simulink model "VectorControl003"  (R2019b)
settings: Solver=ode15s  StartTime=0  StopTime=1  FixedStep=0.001  MaxStep=1e-4  RelTol=1e-6  AbsTol=1e-6  EnableMultiTasking=on
StopFcn:
  | % TNAnalyzexxxPlot
values from neighbouring files (symbols this model uses):
  CurGainError_U = 1 + 0.2*(rand() - 0.5)    [Param000.m]    (also in StartSim.m)
  CurGainError_V = 1 + 0.2*(rand() - 0.5)    [Param000.m]    (also in StartSim.m)
  CurGainError_W = 1 + 0.2*(rand() - 0.5)    [Param000.m]    (also in StartSim.m)
  CurOfsError_U = 0.5 * rand()    [Param000.m]    (also in StartSim.m = AmpNoise * rand())
  CurOfsError_V = 0.5 * rand()    [Param000.m]    (also in StartSim.m = AmpNoise * rand())
  CurOfsError_W = 0.5 * rand()    [Param000.m]    (also in StartSim.m = AmpNoise * rand())
  DCVoltage = 100    [Param000.m]    (also in StartSim.m; StartSim_NoNoise.m)
  ElecAngOfsError = pi*2.0*(rand() - 0.5)    [Param000.m]    (also in StartSim.m = pi * 2.0 * (rand() - 0.5); StartSim_NoNoise.m = pi * 2.0 * (rand() - 0.5))
  MotInertia = 10*rand()*1e-3    [Param000.m]    (also in StartSim.m = 0.1*rand()*1e-3; StartSim_NoNoise.m = 0.1*rand()*1e-3)
  MotPhaseL = 38.7e-6    (= 3.87e-05)    [Param000.m]    (also in StartSim.m = (0.001 + 10 * rand())*1e-3; StartSim_NoNoise.m = (0.001 + 10 * rand())*1e-3)
  MotPhaseR = 25e-3    (= 0.025)    [Param000.m]    (also in StartSim.m = 0.001 + 10 * rand(); StartSim_NoNoise.m = 0.001 + 10 * rand())
  MotPole = 20    [Param000.m]    (also in StartSim.m = 1; StartSim_NoNoise.m = 1)
  MotVisco = rand()*1e-6    [Param000.m]    (also in StartSim.m = 0.01*rand()*1e-6; StartSim_NoNoise.m = 0.01*rand()*1e-6)
  Ts = 1e-6    (= 1e-06)    [StartSim.m]    (also in StartSim_NoNoise.m)
libraries: powerlib x16, simulink x4, powerlib_meascontrol x2, eePwmGeneratorTwoLevel x1
Description:
  | This example illustrates use of the BLDC in a closed-loop
  | speed and voltage control on a 1 kW, 3000 rpm industrial motor
  | 
  | 
  | Copyright 2008-2017 The MathWorks, Inc.
settings Model: ExtModeAutoUpdateStatusClock=off  Creator=MathWorks  LastModifiedBy=nb1e4
settings SolverCC: AutoScaleAbsTol=off  MaxConsecutiveZCs=10000  ZeroCrossAlgorithm=Adaptive  DecoupledContinuousIntegration=on
settings DataIOCC: Decimation=100  SaveFormat=Array  SignalLoggingName=sigsOut
settings OptimizationCC: DefaultParameterBehavior=Inlined  UseDivisionForNetSlopeComputation=on  UseFloatMulNetSlope=on  InlineInvariantSignals=on  PassReuseOutputArgsAs=Individual arguments  ExpressionDepthLimit=2147483647  ZeroExternalMemoryAtStartup=off  ZeroInternalMemoryAtStartup=off  NoFixptDivByZeroProtection=on  EfficientFloat2IntCast=on  LifeSpan=1  OptimizeDataStoreBuffers=off  BusAssignmentInplaceUpdate=off  OptimizationLevel=level0  EfficientTunableParamExpr=on
settings DebuggingCC: AlgebraicLoopMsg=none  UnderspecifiedInitializationDetection=Classic  MergeDetectMultiDrivingBlocksExec=none  SignalResolutionControl=TryResolveAllWithWarning  MultiTaskDSMMsg=warning  MultiTaskCondExecSysMsg=none  ParameterTunabilityLossMsg=error  FcnCallInpInsideContextMsg=warning  StateNameClashWarn=warning  SFUnexpectedBacktrackingDiag=warning  SFNoUnconditionalDefaultTransitionDiag=warning  SFExecutionAtInitializationDiag=none  ArithmeticOperatorsInVariantConditions=warning
settings HardwareCC: ProdBitPerPointer=32  ProdBitPerSizeT=32  ProdBitPerPtrDiffT=32  ProdLargestAtomicInteger=Long  ProdWordSize=32  ProdLongLongMode=on  ProdHWDeviceType=ARM Compatible->ARM 10  TargetUnknown=on
settings ModelReferenceCC: PropagateSignalLabelsOutOfModel=off
settings SFSimCC: SimUseLocalCustomCode=off  MATLABDynamicMemAlloc=off  CustomCodeUndefinedFunction=UseInterfaceOnly
settings RTWCC: SystemTargetFile=ert.tlc  TemplateMakefile=ert_default_tmf  GenerateReport=on  RTWUseLocalCustomCode=off  IncludeHyperlinkInReport=on  LaunchReport=on  GenerateTraceInfo=on  GenerateTraceReport=on  GenerateTraceReportSl=on  GenerateTraceReportSf=on  GenerateTraceReportEml=on  GenerateCodeMetricsReport=on
settings CodeAppCC: ForceParamTrailComments=on  IgnoreCustomStorageClasses=off  OperatorAnnotations=on  SimulinkDataObjDesc=on  SFDataObjDesc=on  CustomSymbolStrGlobalVar=rt$N$M  CustomSymbolStrType=$N$M  CustomSymbolStrFcn=$N$M$F  CustomSymbolStrMacro=$N$M  InsertBlockDesc=on
settings ERTTargetCC: GenerateSampleERTMain=on  IncludeMdlTerminateFcn=off  CombineSignalStateStructs=on  SupportComplex=off  SupportContinuousTime=on  SupportNonInlinedSFcns=on  InlinedParameterPlacement=NonHierarchical  ERTCustomFileTemplate=example_file_process.tlc  ERTFilePackagingFormat=CompactWithDataFile
settings ConfigComp: CovMetricSettings=dw  CovHtmlReporting=on  CovSaveCumulativeToWorkspaceVar=on  CovSaveSingleToWorkspaceVar=on  CovExternalEMLEnable=off  CovSFcnEnable=off
settings SimscapeCC: SimscapeNormalizeSystem=off

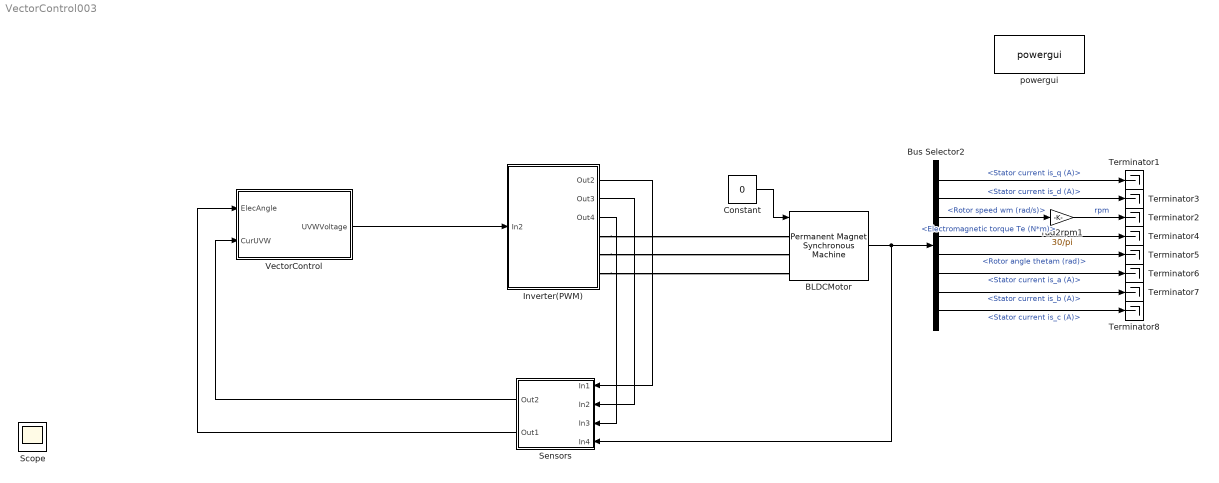
== system VectorControl003 ==
  BLDCMotor : powerlib/Machines/Permanent Magnet Synchronous Machine  NbPhases=3  FluxDistribution=Sinusoidal  RotorType=Round  MechanicalLoad=Torque Tm  PresetModel=No  ShowDetailedParameters=on  MeasurementBus=off  Resistance=MotPhaseR  Inductance=MotPhaseL  dqInductances=[8.5e-3, 8.5e-3]  La=MotPhaseL  MachineConstant=Voltage Constant (V_peak L-L / krpm)  Flux=0.01021  VoltageCst=MotVoltageConst  TorqueCst=0.30629  Flat=120  Mechanical=[MotInertia MotVisco MotPole 0]  PolePairs=20  InitialConditions=[0,0, 0,0]  InitialConditions5ph=[0 0 0 0 0 0]  RefAngle=90 degrees behind phase A axis (modified Park)  IterativeDiscreteModel=Trapezoidal non iterative  TsBlock=-1  TsPowergui=0
  Bus Selector2 : BusSelector  OutputSignals=Stator current is_q (A),Stator current is_d (A),Rotor speed wm (rad/s),Electromagnetic torque Te (N*m),Rotor angle thetam (rad),Stator current is_a (A),Stator current is_b (A),Stator current is_c (A)
  Constant : Constant  Value=0
  Inverter(PWM) : Subsystem
  Sensors : Subsystem
  Terminator{1..8} (8 alike) : Terminator
  VectorControl : Subsystem
  powergui : powerlib/powergui  Priority=2  SimulationMode=Continuous  SampleTime=Ts  frequency=60  Iterations=50  frequencyindice=0  Pbase=100e6  ErrMax=1e-4  UnitsV=kV  UnitsW=MW  buscounter=0  FunctionMessages=off  echomessages=off  EnableUseOfTLC=off  CurrentSourceSwitches=off  DisableSnubberDevices=off  DisableRonSwitches=off  DisableVfSwitches=off  DisplayEquations=off  AutomaticDiscreteSolvers=off  SolverType=Tustin/Backward Euler (TBE)  Interpol=off  ExternalGateDelay=off  methode=off  Ts=100  x0status=blocks  SPID=off  SwTol=0  HookPort=off  NonlinearTolerance=1e-4  nMaxIteration=100  ContinueOnMaxIteration=off  RestoreLinks=warning  ResistiveCurrentMeasurement=off  Frange=[0:2:500]  Ylog=off  Xlog=on  ShowGrid=off  save=off  variable=ZData  structure=0  ZoomFFT=on  StartTime=0.0  cycles=1  DisplayStyle=1  fundamental=60  FreqAxis=off  MaxFrequency=1000  frequencyindicesteady=1  RmsSteady=1  display=off
      settings: SourceProductName=Simscape Electrical
  rad2rpm1 : Gain  Gain=30/pi
  Scope : Scope
  wires:
  Bus Selector2/3 -> rad2rpm1/1  "<Rotor speed wm (rad/s)>"
  BLDCMotor/1 -> Sensors/4(In4), Bus Selector2/1
  rad2rpm1/1 -> Terminator2/1  "rpm"
  Bus Selector2/1 -> Terminator1/1  "<Stator current is_q (A)>"
  Bus Selector2/2 -> Terminator3/1  "<Stator current is_d (A)>"
  Bus Selector2/4 -> Terminator4/1  "<Electromagnetic torque Te (N*m)>"
  Bus Selector2/5 -> Terminator5/1  "<Rotor angle thetam (rad)>"
  Bus Selector2/6 -> Terminator6/1  "<Stator current is_a (A)>"
  Bus Selector2/7 -> Terminator7/1  "<Stator current is_b (A)>"
  Bus Selector2/8 -> Terminator8/1  "<Stator current is_c (A)>"
  Inverter(PWM)/1(Out2) -> Sensors/1(In1)
  Inverter(PWM)/2(Out3) -> Sensors/2(In2)
  Inverter(PWM)/3(Out4) -> Sensors/3(In3)
  VectorControl/1(UVWVoltage) -> Inverter(PWM)/1(In2)
  Sensors/1(Out2) -> VectorControl/2(CurUVW)
  Sensors/2(Out1) -> VectorControl/1(ElecAngle)
  Constant/1 -> BLDCMotor/1
  connections:
  Inverter(PWM)/RConn2 -- BLDCMotor/LConn2
  Inverter(PWM)/RConn3 -- BLDCMotor/LConn3
  Inverter(PWM)/RConn1 -- BLDCMotor/LConn1

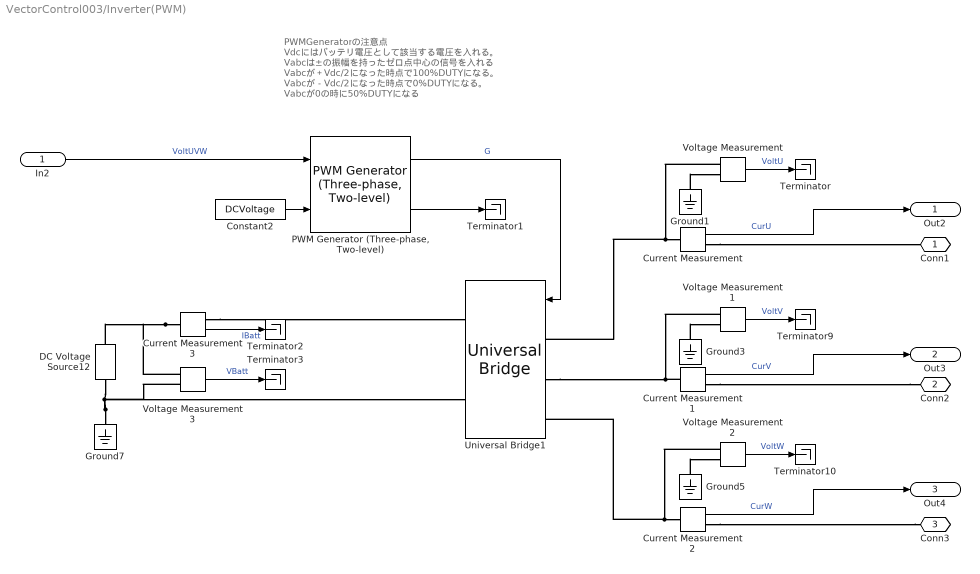
== system VectorControl003/Inverter(PWM) ==
  note: PWMGeneratorの注意点
      | Vdcにはバッテリ電圧として該当する電圧を入れる。
      | Vabcは±の振幅を持ったゼロ点中心の信号を入れる
      | Vabcが＋Vdc/2になった時点で100%DUTYになる。
      | Vabcが－Vdc/2になった時点で0%DUTYになる。
      | Vabcが0の時に50%DUTYになる
  In2 : Inport
  Constant2 : Constant  Value=DCVoltage
  Current Measurement{,1..3} (4 alike) : powerlib/Measurements/Current Measurement  PhasorSimulation=off  OutputType=Complex  PSBequivalent=0
      settings: SourceProductName=Simscape Electrical
  DC Voltage Source12 : powerlib/Electrical Sources/DC Voltage Source  Amplitude=DCVoltage  Measurements=None
      settings: SourceProductName=Simscape Electrical
  Ground{1,3,5,7} (4 alike) : powerlib/Elements/Ground  LConnTagsString=a
      settings: SourceProductName=Simscape Electrical
  "PWM Generator (Three-phase, Two-level)" : eePwmGeneratorTwoLevel/PWM Generator (Three-phase, Two-level)  PWMMode=Continuous PWM (CPWM)  CPWMMode=SPWM: sinusoidal PWM  DPWMMode=60 DPWM: 60 degree discontinuous PWM  fsw=AmpCarryFreq  Ts=1e-6
      settings: SourceProductName=Simscape Electrical  SourceProductBaseCode=PS
  Terminator{,1..3,9..10} (6 alike) : Terminator
  Universal Bridge1 : powerlib/Power Electronics/Universal Bridge  Arms=3  SnubberResistance=1e5  SnubberCapacitance=inf  Device=MOSFET / Diodes  Ron=1e-6  Lon=0  ForwardVoltages="[  0  0  ]"  ForwardVoltage=0  GTOparameters=[ 10e-6 , 20e-6 ]  IGBTparameters=[ 1e-6 , 2e-6 ]  Measurements=None  Measurements_2=None  converterType=Rectifier
      settings: SourceProductName=Simscape Electrical
  Voltage Measurement{,1..3} (4 alike) : powerlib/Measurements/Voltage Measurement  PhasorSimulation=off  OutputType=Complex  PSBequivalent=0
      settings: SourceProductName=Simscape Electrical
  Conn1 : PMIOPort  Side=Right
  Conn2 : PMIOPort  Port=2  Side=Right
  Conn3 : PMIOPort  Port=3  Side=Right
  Out2 : Outport  VectorParamsAs1DForOutWhenUnconnected=off
  Out3 : Outport  Port=2  VectorParamsAs1DForOutWhenUnconnected=off
  Out4 : Outport  Port=3  VectorParamsAs1DForOutWhenUnconnected=off
  wires:
  Voltage Measurement1/1 -> Terminator9/1  "VoltV"
  Voltage Measurement2/1 -> Terminator10/1  "VoltW"
  Voltage Measurement/1 -> Terminator/1  "VoltU"
  Current Measurement1/1 -> Out3/1  "CurV"
  Current Measurement2/1 -> Out4/1  "CurW"
  Current Measurement/1 -> Out2/1  "CurU"
  Current Measurement3/1 -> Terminator2/1  "IBatt"
  Voltage Measurement3/1 -> Terminator3/1  "VBatt"
  Constant2/1 -> "PWM Generator (Three-phase, Two-level)"/2
  "PWM Generator (Three-phase, Two-level)"/1 -> Universal Bridge1/1  "G"
  "PWM Generator (Three-phase, Two-level)"/2 -> Terminator1/1
  In2/1 -> "PWM Generator (Three-phase, Two-level)"/1  "VoltUVW"
  connections:
  Voltage Measurement/LConn1 -- Current Measurement/LConn1 -- Universal Bridge1/LConn1
  Voltage Measurement2/LConn1 -- Current Measurement2/LConn1 -- Universal Bridge1/LConn3
  Current Measurement1/LConn1 -- Voltage Measurement1/LConn1 -- Universal Bridge1/LConn2
  Ground1/LConn1 -- Voltage Measurement/LConn2
  Ground3/LConn1 -- Voltage Measurement1/LConn2
  Ground5/LConn1 -- Voltage Measurement2/LConn2
  Current Measurement3/LConn1 -- Voltage Measurement3/LConn1 -- DC Voltage Source12/RConn1
  Ground7/LConn1 -- Universal Bridge1/RConn2 -- Voltage Measurement3/LConn2 -- DC Voltage Source12/LConn1
  Current Measurement/RConn1 -- Conn1/RConn1
  Current Measurement1/RConn1 -- Conn2/RConn1
  Current Measurement2/RConn1 -- Conn3/RConn1
  Current Measurement3/RConn1 -- Universal Bridge1/RConn1

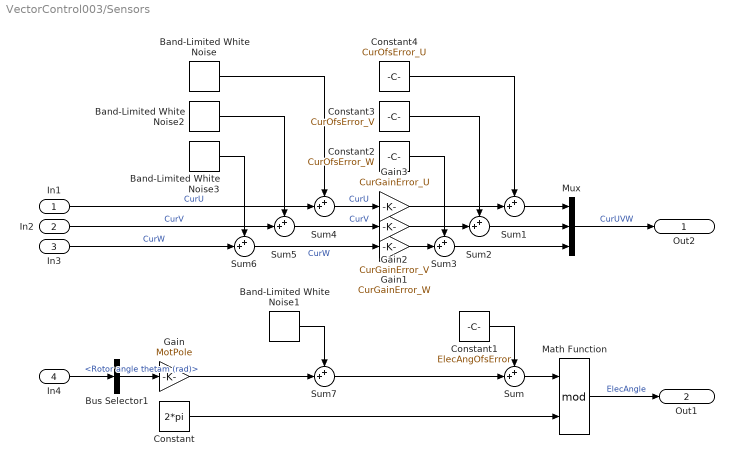
== system VectorControl003/Sensors ==
  In1 : Inport
  In2 : Inport  Port=2
  In3 : Inport  Port=3
  In4 : Inport  Port=4
  Band-Limited White Noise : simulink/Sources/Band-Limited White Noise  Cov=CurNoise  Ts=1e-6  seed=[23341]
  Band-Limited White Noise1 : simulink/Sources/Band-Limited White Noise  Cov=ElecAngNoise  Ts=1e-6  seed=[23344]
  Band-Limited White Noise2 : simulink/Sources/Band-Limited White Noise  Cov=CurNoise  Ts=1e-6  seed=[23342]
  Band-Limited White Noise3 : simulink/Sources/Band-Limited White Noise  Cov=1e-9  Ts=1e-6  seed=[23343]
  Bus Selector1 : BusSelector  OutputSignals=Rotor angle thetam (rad)
  Constant : Constant  Value=2*pi
  Constant1 : Constant  Value=ElecAngOfsError
  Constant2 : Constant  Value=CurOfsError_W
  Constant3 : Constant  Value=CurOfsError_V
  Constant4 : Constant  Value=CurOfsError_U
  Gain : Gain  Gain=MotPole
  Gain1 : Gain  Gain=CurGainError_W
  Gain2 : Gain  Gain=CurGainError_V
  Gain3 : Gain  Gain=CurGainError_U
  Math Function : Math  Operator=mod  SaturateOnIntegerOverflow=on
  Mux : Mux  Inputs=3
  Sum{,1..7} (8 alike) : Sum  Inputs=++|
  Out2 : Outport  VectorParamsAs1DForOutWhenUnconnected=off
  Out1 : Outport  Port=2  VectorParamsAs1DForOutWhenUnconnected=off
  wires:
  Sum7/1 -> Sum/2
  Bus Selector1/1 -> Gain/1  "<Rotor angle thetam (rad)>"
  Sum6/1 -> Gain1/1  "CurW"
  Sum4/1 -> Gain3/1  "CurU"
  In4/1 -> Bus Selector1/1
  Constant/1 -> Math Function/2
  Sum5/1 -> Gain2/1  "CurV"
  Math Function/1 -> Out1/1  "ElecAngle"
  Mux/1 -> Out2/1  "CurUVW"
  Sum/1 -> Math Function/1
  Constant1/1 -> Sum/1
  Gain3/1 -> Sum1/2
  Sum2/1 -> Mux/2
  Sum3/1 -> Mux/3
  Sum1/1 -> Mux/1
  Gain2/1 -> Sum2/2
  Gain1/1 -> Sum3/2
  Constant4/1 -> Sum1/1
  Constant3/1 -> Sum2/1
  Constant2/1 -> Sum3/1
  In1/1 -> Sum4/2  "CurU"
  In2/1 -> Sum5/2  "CurV"
  In3/1 -> Sum6/2  "CurW"
  Gain/1 -> Sum7/2
  Band-Limited White Noise1/1 -> Sum7/1
  Band-Limited White Noise/1 -> Sum4/1
  Band-Limited White Noise2/1 -> Sum5/1
  Band-Limited White Noise3/1 -> Sum6/1

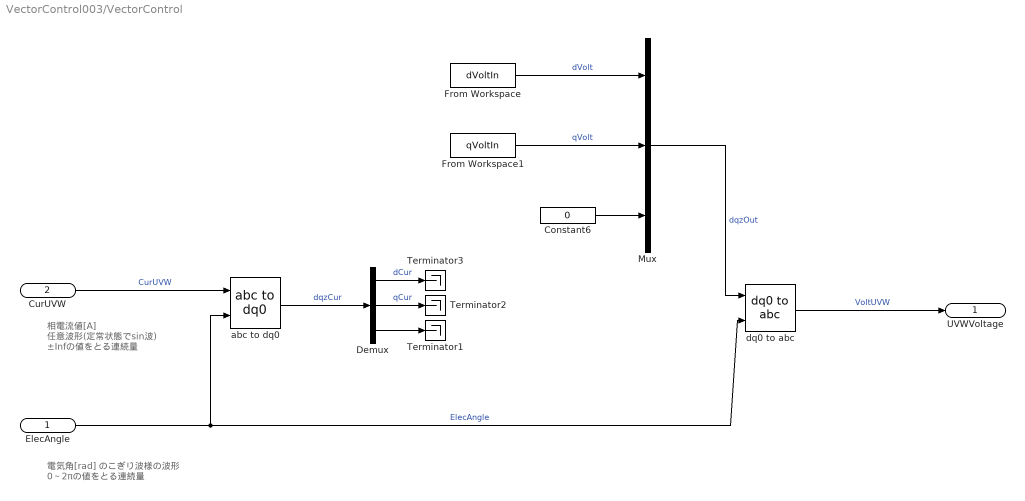
== system VectorControl003/VectorControl ==
  note: 電気角[rad]
      | のこぎり波様の波形
      | 0～2πの値をとる連続量
  note: 相電流値[A]
      | 任意波形(定常状態でsin波)
      | ±Infの値をとる連続量
  ElecAngle : Inport
  CurUVW : Inport  Port=2
  Constant6 : Constant  Value=0
  Demux : Demux  Outputs=3
  From Workspace : FromWorkspace  VariableName=dVoltIn  SampleTime=0
  From Workspace1 : FromWorkspace  VariableName=qVoltIn  SampleTime=0
  Mux : Mux  Inputs=3
  Terminator1 : Terminator
  Terminator2 : Terminator
  Terminator3 : Terminator
  abc to dq0 : powerlib_meascontrol/Transformations/abc to dq0  Alignment=90 degrees behind phase A axis
      settings: SourceProductName=Simscape Electrical
  dq0 to abc : powerlib_meascontrol/Transformations/dq0 to abc  Alignment=90 degrees behind phase A axis
      settings: SourceProductName=Simscape Electrical
  UVWVoltage : Outport  VectorParamsAs1DForOutWhenUnconnected=off
  wires:
  ElecAngle/1 -> dq0 to abc/2, abc to dq0/2  "ElecAngle"
  dq0 to abc/1 -> UVWVoltage/1  "VoltUVW"
  abc to dq0/1 -> Demux/1  "dqzCur"
  Mux/1 -> dq0 to abc/1  "dqzOut"
  Constant6/1 -> Mux/3
  Demux/3 -> Terminator1/1
  CurUVW/1 -> abc to dq0/1  "CurUVW"
  Demux/1 -> Terminator3/1  "dCur"
  Demux/2 -> Terminator2/1  "qCur"
  From Workspace/1 -> Mux/1  "dVolt"
  From Workspace1/1 -> Mux/2  "qVolt"
